simulink model "QuadModel"  (R2022b)
settings: Solver=VariableStepAuto  StartTime=0.0  StopTime=50  RelTol=1e-3  AbsTol=1e-3  EnableMultiTasking=on
undefined symbols (not defined in the file): Ixx, Iyy, Izz, k, mass, prD, prI, prP, X, Y, Z, zD, zI, zP
libraries: sm_lib x42, nesl_utility x35, slpidlib x4
(part 3 of 3)

== matlab function QuadModel/Drone Plant/MATLAB Function1 ==
  data: u input; beta output
function beta = fcn(u)

beta = 180*u(2)/pi;
